simulink model "servo"  (R2018a)
settings: Solver=FixedStepAuto  StartTime=0.0  StopTime=1  FixedStep=0.005  RelTol=1e-3
libraries: aerolibactuator x2
settings Model: Creator=mengc  LastModifiedBy=mengc

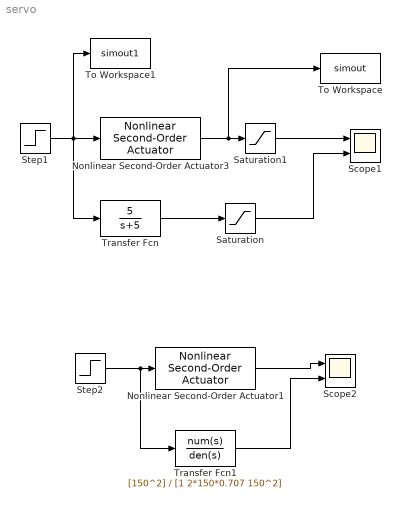
== system servo ==
  Nonlinear Second-Order Actuator1 : aerolibactuator/Nonlinear Second-Order Actuator  wn_fin=100  z_fin=1  fin_max=500  fin_min=-500  fin_maxrate=1000  fin_act_0=0  fin_act_vel=0
      settings: SourceProductName=Aerospace Blockset  SourceProductBaseCode=AE
  Nonlinear Second-Order Actuator3 : aerolibactuator/Nonlinear Second-Order Actuator  wn_fin=50  z_fin=1  fin_max=500  fin_min=-500  fin_maxrate=1000  fin_act_0=0  fin_act_vel=0
      settings: SourceProductName=Aerospace Blockset  SourceProductBaseCode=AE
  Saturation : Saturate  UpperLimit=500  LowerLimit=-500
  Saturation1 : Saturate  UpperLimit=500  LowerLimit=-500
  Scope1 : Scope  NumInputPorts=2
  Scope2 : Scope  NumInputPorts=2
  Step1 : Step  Time=0.1  After=400  SampleTime=0
  Step2 : Step  Time=0.1  After=0.1  SampleTime=0
  To Workspace : ToWorkspace  VariableName=simout  SaveFormat=Timeseries  SampleTime=-1
  To Workspace1 : ToWorkspace  VariableName=simout1  SaveFormat=Timeseries  SampleTime=-1
  Transfer Fcn : TransferFcn  Numerator=[5]  Denominator=[1 5]
  Transfer Fcn1 : TransferFcn  Numerator=[150^2]  Denominator=[1 2*150*0.707 150^2]
  wires:
  Step1/1 -> Nonlinear Second-Order Actuator3/1, Transfer Fcn/1, To Workspace1/1
  Nonlinear Second-Order Actuator3/1 -> To Workspace/1, Saturation1/1
  Transfer Fcn/1 -> Saturation/1
  Transfer Fcn1/1 -> Scope2/2
  Step2/1 -> Transfer Fcn1/1, Nonlinear Second-Order Actuator1/1
  Nonlinear Second-Order Actuator1/1 -> Scope2/1
  Saturation1/1 -> Scope1/1
  Saturation/1 -> Scope1/2
